simulink model "determinacao_indireta_comparacao"  (Simulink 7.9)
settings: Solver=ode45  StartTime=0.0  StopTime=10.0  RelTol=1e-3
settings Model: Creator=Danilo  LastModifiedBy=Danilo

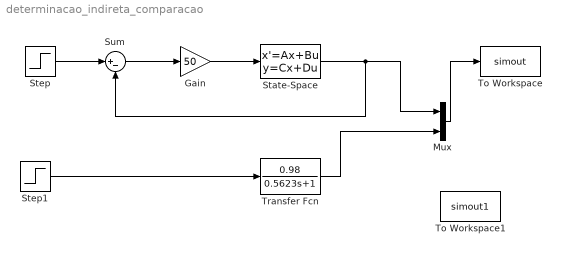
== system determinacao_indireta_comparacao ==
  Gain : Gain  Gain=50
  Mux : Mux  Inputs=2
  State-Space : StateSpace  A=-0.03  C=0.0333  D=0
  Step : Step  Time=0  SampleTime=0
  Step1 : Step  Time=0  SampleTime=0
  Sum : Sum  Inputs=|+-
  To Workspace : ToWorkspace  VariableName=simout  SampleTime=-1
  To Workspace1 : ToWorkspace  VariableName=simout1  SampleTime=-1
  Transfer Fcn : TransferFcn  Numerator=[0.98]  Denominator=[0.5623 1]
  wires:
  State-Space/1 -> Sum/2, Mux/1
  Gain/1 -> State-Space/1
  Step/1 -> Sum/1
  Sum/1 -> Gain/1
  Transfer Fcn/1 -> Mux/2
  Step1/1 -> Transfer Fcn/1
  Mux/1 -> To Workspace/1
